simulink model "DatasVerificacion"  (R2020a)
settings: Solver=VariableStepAuto  StartTime=0.0  StopTime=15  RelTol=1e-3
settings Model: Creator=HP  LastModifiedBy=HP

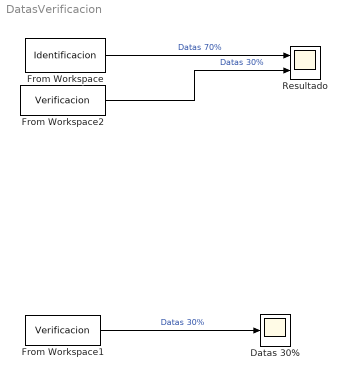
== system DatasVerificacion ==
  Datas 30% : Scope
  From Workspace : FromWorkspace  VariableName=Identificacion
  From Workspace1 : FromWorkspace  VariableName=Verificacion
  From Workspace2 : FromWorkspace  VariableName=Verificacion
  Resultado : Scope  NumInputPorts=2
  wires:
  From Workspace/1 -> Resultado/1  "Datas 70%"
  From Workspace1/1 -> Datas 30%/1  "Datas 30%"
  From Workspace2/1 -> Resultado/2  "Datas 30%"
